simulink model "plantPWM"  (R2018a)
settings: Solver=ode15s  StartTime=0.0  StopTime=10.0  RelTol=1e-3  EnableMultiTasking=on
PreLoadFcn:
  | etc_plant_data;
  | Fs = 1000;
values from neighbouring files (symbols this model uses):
  J = 0.000245    [allParamValues.mat]
libraries: simulink x1
settings Model: Creator=nicholas  LastModifiedBy=bneiswan
settings SolverCC: MaxConsecutiveZCs=25
settings DataIOCC: LimitDataPoints=on  SaveFormat=Array
settings OptimizationCC: DefaultParameterBehavior=Inlined  ExpressionDepthLimit=2147483647  InitFltsAndDblsToZero=on  LifeSpan=inf
settings DebuggingCC: UnderspecifiedInitializationDetection=Classic  MergeDetectMultiDrivingBlocksExec=none  ParameterPrecisionLossMsg=none  FcnCallInpInsideContextMsg=warning  AllowSymbolicDim=off  StateNameClashWarn=warning  SFUnexpectedBacktrackingDiag=warning  SFNoUnconditionalDefaultTransitionDiag=warning  SFExecutionAtInitializationDiag=none
settings HardwareCC: ProdBitPerPointer=32  ProdBitPerSizeT=32  ProdBitPerPtrDiffT=32  ProdLargestAtomicFloat=None  ProdIntDivRoundTo=Undefined  ProdEndianess=Unspecified  ProdWordSize=32  ProdHWDeviceType=32-bit Generic
settings ModelReferenceCC: ModelReferenceMinAlgLoopOccurrences=on  PropagateSignalLabelsOutOfModel=off
settings CodeAppCC: StateflowObjectComments=on
settings GRTTargetCC: TargetLangStandard=C89/C90 (ANSI)  GeneratePreprocessorConditionals=Disable all  CombineOutputUpdateFcns=off  GRTInterface=on
settings ConfigComp: CovMetricSettings=dw  CovHtmlReporting=on  CovSaveCumulativeToWorkspaceVar=on  CovSaveSingleToWorkspaceVar=on  CovExternalEMLEnable=off  CovSFcnEnable=off

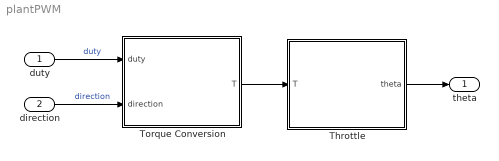
== system plantPWM ==
  duty : Inport
  direction : Inport  Port=2
  Throttle : Subsystem
  Torque Conversion : Subsystem
  theta : Outport
  wires:
  duty/1 -> Torque Conversion/1(duty)  "duty"
  direction/1 -> Torque Conversion/2(direction)  "direction"
  Torque Conversion/1(T) -> Throttle/1(T)
  Throttle/1(theta) -> theta/1

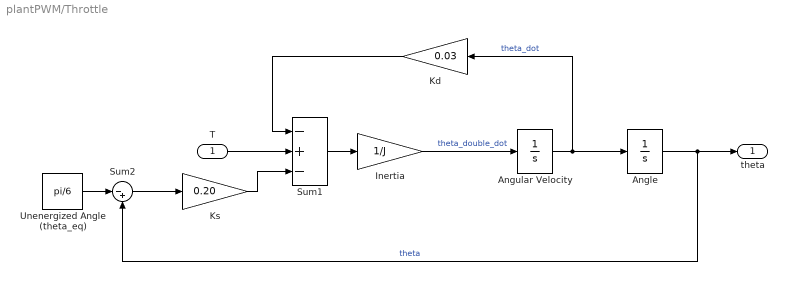
== system plantPWM/Throttle ==
  T : Inport
  Angle : Integrator  InitialCondition=pi/6  LimitOutput=on  UpperSaturationLimit=pi/2  LowerSaturationLimit=0
      settings: AttributesFormatString=Initial condition: %<InitialCondition>\n%<LowerSaturationLimit> <= theta <= %<UpperSaturationLimit>
  Angular Velocity : Integrator
      settings: AttributesFormatString=Initial condition: %<InitialCondition>
  Inertia : Gain  Gain=1/J  SaturateOnIntegerOverflow=on  OutDataTypeStr=Inherit: Same as input  ParamDataTypeStr=Inherit: Same as input
  Kd : Gain  Gain=0.03  SaturateOnIntegerOverflow=on  OutDataTypeStr=Inherit: Same as input  ParamDataTypeStr=Inherit: Same as input
  Ks : Gain  Gain=0.20  SaturateOnIntegerOverflow=on  OutDataTypeStr=Inherit: Same as input  ParamDataTypeStr=Inherit: Same as input
  Sum1 : Sum  Inputs=-+-  SaturateOnIntegerOverflow=on
  Sum2 : Sum  Inputs=|-+  SaturateOnIntegerOverflow=on
  Unenergized Angle (theta_eq) : Constant  Value=pi/6
  theta : Outport
  wires:
  Sum1/1 -> Inertia/1
  Inertia/1 -> Angular Velocity/1  "theta_double_dot"
  Kd/1 -> Sum1/1
  Sum2/1 -> Ks/1
  Ks/1 -> Sum1/3
  Unenergized Angle (theta_eq)/1 -> Sum2/1
  Angle/1 -> theta/1, Sum2/2  "theta"
  Angular Velocity/1 -> Angle/1, Kd/1  "theta_dot"
  T/1 -> Sum1/2

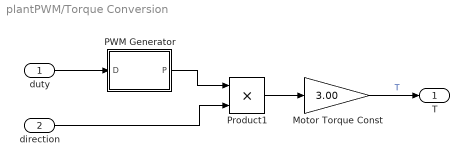
== system plantPWM/Torque Conversion ==
  duty : Inport
  direction : Inport  Port=2
  Motor Torque Const : Gain  Gain=3.00  SaturateOnIntegerOverflow=on  OutDataTypeStr=Inherit: Same as input  ParamDataTypeStr=Inherit: Same as input
  PWM Generator : Subsystem  DialogController=POWERSYS.PowerSysDialog
  Product1 : Product  SaturateOnIntegerOverflow=on  OutDataTypeStr=Inherit: Same as first input
  T : Outport
  wires:
  duty/1 -> PWM Generator/1(D)
  Motor Torque Const/1 -> T/1  "T"
  direction/1 -> Product1/2
  Product1/1 -> Motor Torque Const/1
  PWM Generator/1(P) -> Product1/1

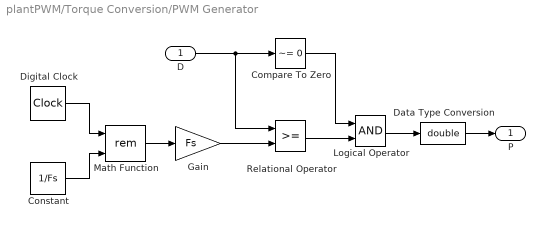
== system plantPWM/Torque Conversion/PWM Generator ==
  D : Inport
  Compare To Zero : simulink/Logic and Bit Operations/Compare To Zero  relop=~=  OutDataTypeStr=boolean
  Constant : Constant  Value=1/Fs  SampleTime=0
  Data Type Conversion : DataTypeConversion  OutDataTypeStr=double
  Digital Clock : DigitalClock  SampleTime=1/(50*Fs)
      settings: AttributesFormatString=Ts = %<SampleTime>
  Gain : Gain  Gain=Fs  SaturateOnIntegerOverflow=on  OutDataTypeStr=Inherit: Same as input  ParamDataTypeStr=Inherit: Same as input
  Logical Operator : Logic  AllPortsSameDT=off  OutDataTypeStr=boolean
  Math Function : Math  Operator=rem  SaturateOnIntegerOverflow=on
  Relational Operator : RelationalOperator  OutDataTypeStr=boolean  RndMeth=Nearest
  P : Outport
  wires:
  D/1 -> Compare To Zero/1, Relational Operator/1
  Relational Operator/1 -> Logical Operator/2
  Compare To Zero/1 -> Logical Operator/1
  Logical Operator/1 -> Data Type Conversion/1
  Data Type Conversion/1 -> P/1
  Gain/1 -> Relational Operator/2
  Math Function/1 -> Gain/1
  Constant/1 -> Math Function/2
  Digital Clock/1 -> Math Function/1
